simulink model "rerer"  (R2020b)
settings: Solver=ode45  StartTime=0.0  StopTime=10.0  RelTol=1e-3
settings Model: Creator=반달  LastModifiedBy=반달
settings DataIOCC: ReturnWorkspaceOutputs=off

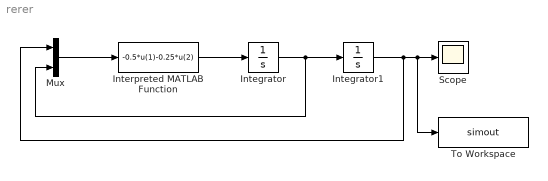
== system rerer ==
  Integrator : Integrator  InitialCondition=6
  Integrator1 : Integrator  InitialCondition=4
  Interpreted MATLAB Function : MATLABFcn  MATLABFcn=-0.5*u(1)-0.25*u(2)
  Mux : Mux  Inputs=2
  Scope : Scope
  To Workspace : ToWorkspace  VariableName=simout  SaveFormat=Structure With Time  SampleTime=-1
  wires:
  Interpreted MATLAB Function/1 -> Integrator/1
  Mux/1 -> Interpreted MATLAB Function/1
  Integrator/1 -> Mux/2, Integrator1/1
  Integrator1/1 -> Mux/1, To Workspace/1, Scope/1
